simulink model "test_multirate"  (R2012b)
settings: Solver=FixedStepDiscrete  SolverMode=SingleTasking  StartTime=0.0  StopTime=10.0  FixedStep=0.01  RelTol=1e-3
settings Model: Creator=peselnikmg  LastModifiedBy=peselnikmg
settings DataIOCC: SignalLoggingSaveFormat=ModelDataLogs  SaveOutput=off  SaveTime=off
settings OptimizationCC: InlineParams=on  OptimizeModelRefInitCode=on  LifeSpan=1
settings HardwareCC: ProdBitPerInt=16  ProdBitPerPointer=16  ProdIntDivRoundTo=Zero  ProdEndianess=LittleEndian  ProdWordSize=16  ProdHWDeviceType=Texas Instruments->MSP430
settings RTWCC: SystemTargetFile=launchpad.tlc  TemplateMakefile=launchpad_tmf  Description=TI LaunchPad  GenerateReport=on  ProcessScript=launchpad_make_rtw_hook  IncludeHyperlinkInReport=on  LaunchReport=on  GenerateTraceInfo=on  GenerateTraceReport=on  GenerateTraceReportSl=on  GenerateTraceReportSf=on  GenerateTraceReportEml=on
settings CodeAppCC: IgnoreCustomStorageClasses=off
settings STFCustomTargetCC: CodeReplacementLibrary=ANSI_C  CombineOutputUpdateFcns=on  ERTCustomFileBanners=on  SupportAbsoluteTime=off  SupportNonFinite=off  SupportComplex=off  PurelyIntegerCode=on  SupportContinuousTime=off  SupportNonInlinedSFcns=off  GRTInterface=off  SystemTargetFile=launchpad.tlc
settings ERTTargetCC: CodeReplacementLibrary=ANSI_C  MultiwordLength=2048  ParMdlRefBuildCompliant=off  CompOptLevelCompliant=off  ConcurrentExecutionCompliant=off  ERTFirstTimeCompliant=off  SupportAbsoluteTime=off  SupportNonFinite=off  SupportComplex=off  PurelyIntegerCode=on  ModelStepFunctionPrototypeControlCompliant=off  CPPClassGenCompliant=off  InlinedParameterPlacement=NonHierarchical  ERTCustomFileTemplate=launchpad_srmain.tlc  ConvertIfToSwitch=off  SuppressUnreachableDefaultCases=off

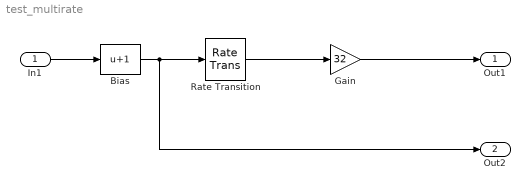
== system test_multirate ==
  In1 : Inport  OutDataTypeStr=int16  PortDimensions=1  SampleTime=[0.01,0]
  Bias : Bias  Bias=1
  Gain : Gain  Gain=32  OutDataTypeStr=int16
  Rate Transition : RateTransition  OutPortSampleTime=0.1
  Out1 : Outport  OutDataTypeStr=int16  PortDimensions=1  SampleTime=[0.10000000000000001,0]
  Out2 : Outport  Port=2  OutDataTypeStr=int16  PortDimensions=1  SampleTime=[0.01,0]
  wires:
  In1/1 -> Bias/1
  Rate Transition/1 -> Gain/1
  Gain/1 -> Out1/1
  Bias/1 -> Rate Transition/1, Out2/1
